simulink model "RCAMsimulation"  (R2022a)
settings: Solver=VariableStepAuto  StartTime=0.0  StopTime=TF  RelTol=1e-3
values from neighbouring files (symbols this model uses):
  x0 = [85 ... (first row only)    [initialize_constants.m]
undefined symbols (not defined in the file or in its folder): RCAM_model
settings Model: Creator=psriva2  LastModifiedBy=psriva2

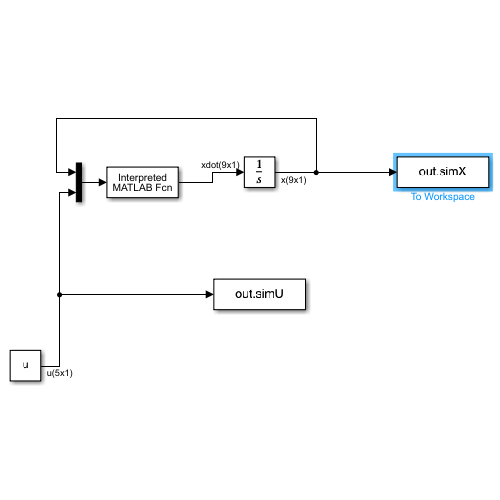
[thumbnail: Simulink's stored preview of the top-level diagram]
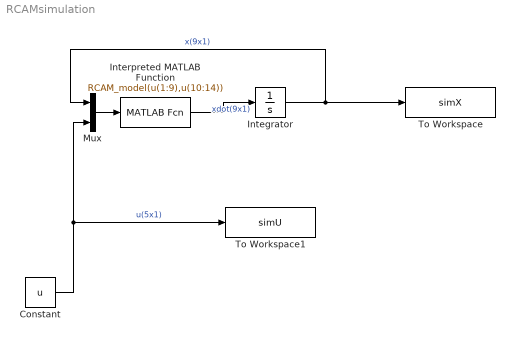
== system RCAMsimulation ==
  Constant : Constant  Value=u
  Integrator : Integrator  InitialCondition=x0
  Interpreted MATLAB Function : MATLABFcn  MATLABFcn=RCAM_model(u(1:9),u(10:14))
  Mux : Mux  Inputs=2
  To Workspace : ToWorkspace  VariableName=simX  SaveFormat=Timeseries  SampleTime=-1
  To Workspace1 : ToWorkspace  VariableName=simU  SaveFormat=Timeseries  SampleTime=-1
  wires:
  Interpreted MATLAB Function/1 -> Integrator/1  "xdot(9x1)"
  Constant/1 -> Mux/2, To Workspace1/1  "u(5x1)"
  Integrator/1 -> Mux/1, To Workspace/1  "x(9x1)"
  Mux/1 -> Interpreted MATLAB Function/1
